simulink model "water_simul"  (R2025b)
settings: Solver=FixedStepAuto  StartTime=0.0  StopTime=3  FixedStep=0.001  RelTol=1e-3
InitFcn:
  | run('rocket3d_params.m')
values from neighbouring files (symbols this model uses):
  A_e = pi*(d_e/2)^2    (= 0.000346360590058)    [rocket3d_params.m]
  beta_poly = 1.31    [rocket3d_params.m]
  C_d_air = 0.90    (= 0.9)    [rocket3d_params.m]
  C_d_water = 0.85    [rocket3d_params.m]
  P_atm = 101325    [rocket3d_params.m]
  P_i = 50*6894.75 + P_atm    (= 446062.5)    [rocket3d_params.m]
  rho_water = 1000    [rocket3d_params.m]
  T_i = T_celsius + 273.15    (= 298.15)    [rocket3d_params.m]
  Ts = 0.001    [rocket3d_params.m]    (also in stability_margin_timehistory.m)
  V_bottle = 1.5e-3    (= 0.0015)    [rocket3d_params.m]
  V_gas_i = V_bottle - V_water_i    (= 0.00092)    [rocket3d_params.m]
undefined symbols (not defined in the file or in its folder): gamma, R
settings Model: Creator=user  LastModifiedBy=user

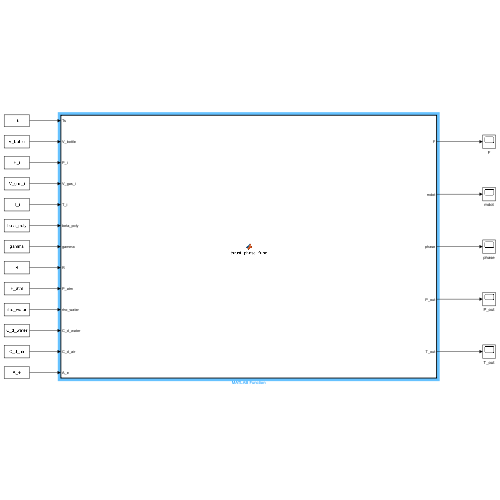
[thumbnail: Simulink's stored preview of the top-level diagram]
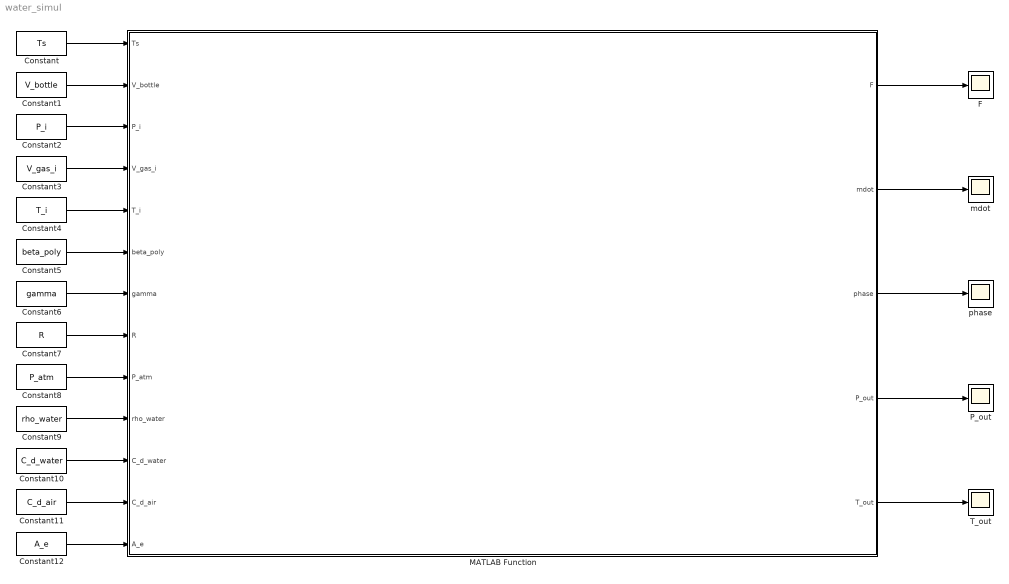
== system water_simul ==
  Constant : Constant  Value=Ts
  Constant1 : Constant  Value=V_bottle
  Constant10 : Constant  Value=C_d_water
  Constant11 : Constant  Value=C_d_air
  Constant12 : Constant  Value=A_e
  Constant2 : Constant  Value=P_i
  Constant3 : Constant  Value=V_gas_i
  Constant4 : Constant  Value=T_i
  Constant5 : Constant  Value=beta_poly
  Constant6 : Constant  Value=gamma
  Constant7 : Constant  Value=R
  Constant8 : Constant  Value=P_atm
  Constant9 : Constant  Value=rho_water
  F : Scope
      settings: ActiveDisplayYMinimum=-21.567254282185612  ActiveDisplayYMaximum=194.10528853967054
  MATLAB Function : MATLAB Function  TreatAsAtomicUnit=on
  P_out : Scope
      settings: ActiveDisplayYMinimum=58232.812500000015  ActiveDisplayYMaximum=489154.6875  DataLoggingVariableName=ScopeData3
  T_out : Scope
      settings: ActiveDisplayYMinimum=190.18723511364928  ActiveDisplayYMaximum=310.14586276515007  DataLoggingVariableName=ScopeData4
  mdot : Scope
      settings: ActiveDisplayYMinimum=-8.6967939527182061  ActiveDisplayYMaximum=0.96631043919091153
  phase : Scope
      settings: ActiveDisplayYMinimum=0.85596730640726482  ActiveDisplayYMaximum=3.1235410025523898  DataLoggingVariableName=ScopeData2
  wires:
  Constant/1 -> MATLAB Function/1(Ts)
  Constant1/1 -> MATLAB Function/2(V_bottle)
  Constant2/1 -> MATLAB Function/3(P_i)
  Constant3/1 -> MATLAB Function/4(V_gas_i)
  Constant4/1 -> MATLAB Function/5(T_i)
  Constant5/1 -> MATLAB Function/6(beta_poly)
  Constant6/1 -> MATLAB Function/7(gamma)
  Constant7/1 -> MATLAB Function/8(R)
  Constant8/1 -> MATLAB Function/9(P_atm)
  Constant9/1 -> MATLAB Function/10(rho_water)
  Constant10/1 -> MATLAB Function/11(C_d_water)
  Constant11/1 -> MATLAB Function/12(C_d_air)
  Constant12/1 -> MATLAB Function/13(A_e)
  MATLAB Function/5(T_out) -> T_out/1
  MATLAB Function/4(P_out) -> P_out/1
  MATLAB Function/3(phase) -> phase/1
  MATLAB Function/2(mdot) -> mdot/1
  MATLAB Function/1(F) -> F/1

== matlab function water_simul/MATLAB Function ==
  data: Ts input; F output; V_bottle input; P_i input; V_gas_i input; T_i input; beta_poly input; gamma input; R input; P_atm input; rho_water input; C_d_water input; C_d_air input; A_e input; mdot output; phase output; P_out output; T_out output
function [F, mdot, phase, P_out, T_out] = thrust_phase_func(Ts, ...
        V_bottle, P_i, V_gas_i, T_i, beta_poly, gamma, R, P_atm, ...
        rho_water, C_d_water, C_d_air, A_e)
%#codegen
% 물로켓 추력 + 질량유량 계산
% (기존 2D 스크립트의 phase 1~3 while문 로직을 한 스텝짜리 함수로 이식)
%
% Simulink "MATLAB Function" 블록에 이 코드를 그대로 붙여넣고,
% 입력은 전부 rocket3d_params.m 의 값을 Constant 블록으로 연결하세요.
% (Ts만 샘플타임이고 나머지는 고정 파라미터입니다.)
%
% 출력
%   F     : 노즐 추력 [N]
%   mdot  : 추진제(물+공기) 질량유량 [kg/s] (분출이므로 음수)
%   phase : 현재 단계 (1=물 분출, 2=공기 분출, 3=탄도비행)
%   P_out, T_out : 내부 압력[Pa] / 온도[K] (로깅·디버깅용)

persistent V_gas P T phase_s P_phase2_i T_phase2_i

if isempty(V_gas)
    V_gas      = V_gas_i;
    P          = P_i;
    T          = T_i;
    phase_s    = uint8(1);
    P_phase2_i = P_i;
    T_phase2_i = T_i;
end

F = 0; mdot = 0;

switch phase_s
    case 1   % 물 분출 (폴리트로픽 압축공기 팽창)
        P = P_i * (V_gas_i / V_gas)^beta_poly;
        if P > P_atm
            v_e  = C_d_water * sqrt(2*(P - P_atm)/rho_water);
            F    = 2 * C_d_water^2 * A_e * (P - P_atm);
            mdot = -rho_water * A_e * v_e;
            V_gas = V_gas + A_e * v_e * Ts;
            if V_gas >= V_bottle
                V_gas      = V_bottle;
                phase_s    = uint8(2);
                P_phase2_i = P;
                T_phase2_i = T_i * (P / P_i)^((beta_poly - 1)/beta_poly);
                T = T_phase2_i;
            end
        else
            phase_s = uint8(2);
        end

    case 2   % 공기 분출 (단열 팽창, choked/subsonic 판정)
        if P > P_atm * 1.01
            T = T_phase2_i * (P / P_phase2_i)^((gamma - 1)/gamma);
            P_crit = 1.893 * P_atm;
            if P >= P_crit
                P_exit   = P * (2/(gamma+1))^(gamma/(gamma-1));
                T_exit   = T * (2/(gamma+1));
                v_exit   = sqrt(gamma * R * T_exit);
                rho_exit = P_exit / (R * T_exit);
                m_mag    = C_d_air * A_e * rho_exit * v_exit;
                F        = m_mag * v_exit + (P_exit - P_atm) * A_e;
                dP_dt    = -(C_d_air*A_e*gamma*P/V_bottle) * ...
                            sqrt(gamma*R*T*(2/(gamma+1))^((gamma+1)/(gamma-1)));
            else
                P_exit   = P_atm;
                v_exit   = sqrt((2*gamma*R*T/(gamma-1)) * (1 - (P_atm/P)^((gamma-1)/gamma)));
                T_exit   = T * (P_atm/P)^((gamma-1)/gamma);
                rho_exit = P_atm / (R * T_exit);
                m_mag    = C_d_air * A_e * rho_exit * v_exit;
                F        = m_mag * v_exit;
                term1 = (P_atm/P)^(2/gamma);
                term2 = (P_atm/P)^((gamma+1)/gamma);
                if term1 > term2
                    dP_dt = -(C_d_air*A_e*gamma*P/V_bottle) * ...
                             sqrt((2*gamma*R*T/(gamma-1)) * (term1 - term2));
                else
                    dP_dt = 0;
                end
            end
            mdot = -m_mag;
            P = P + dP_dt * Ts;
        else
            phase_s = uint8(3);
            P = P_atm;
        end

    case 3   % 탄도비행 (추력 없음)
    P = P_atm; F = 0; mdot = 0;
    k_heat = 5;                          % 대기와의 열교환 계수 (원본과 동일)
    T = T_i + (T - T_i) * exp(-k_heat*Ts);
end

phase = double(phase_s);
P_out = P;
T_out = T;
end
